simulink model "Pacemaker_01"  (R2020a)
settings: Solver=FixedStepAuto  StartTime=0.0  StopTime=10.0  FixedStep=1e-3  RelTol=1e-3  EnableMultiTasking=on
undefined symbols (not defined in the file): D0, D10, D11, D2, D5, D8, PTA0, PTA2, PTB9, PTC16, PTD0, PTD2
libraries: frdmk64flib x14
settings Model: ExtModeTrigDuration=5  Creator=forre  LastModifiedBy=forre
settings OptimizationCC: EnhancedBackFolding=on  PassReuseOutputArgsAs=Individual arguments  ZeroExternalMemoryAtStartup=off  ZeroInternalMemoryAtStartup=off  MaxStackSize=64  OptimizeBlockOrder=speed  DifferentSizesBufferReuse=on  OptimizationCustomize=off  EfficientTunableParamExpr=on
settings DebuggingCC: ParameterTunabilityLossMsg=error
settings HardwareCC: ProdBitPerPointer=32  ProdBitPerSizeT=32  ProdBitPerPtrDiffT=32  ProdLargestAtomicInteger=Long  ProdLargestAtomicFloat=Double  ProdWordSize=32  ProdHWDeviceType=ARM Compatible->ARM Cortex
settings SFSimCC: MATLABDynamicMemAlloc=off
settings RTWCC: SystemTargetFile=ert.tlc  HardwareBoard=NXP FRDM-K64F  TemplateMakefile=ert_default_tmf  Toolchain=GNU Tools for ARM Embedded Processors
settings CodeAppCC: ForceParamTrailComments=on  IgnoreCustomStorageClasses=off  OperatorAnnotations=on  SimulinkDataObjDesc=on  SFDataObjDesc=on  InsertBlockDesc=on

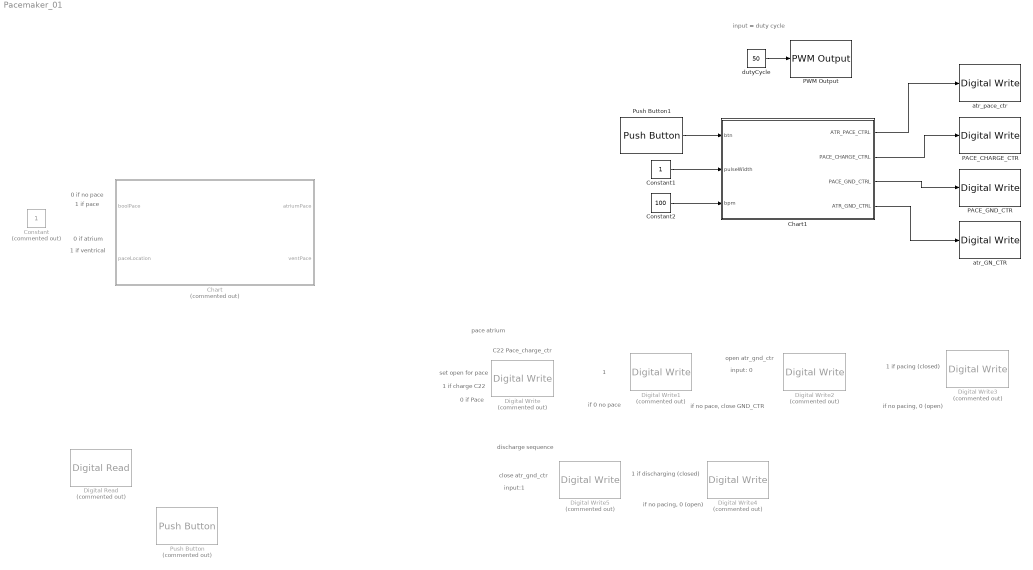
== system Pacemaker_01 ==
  note: 1 if pace
  note: 0 if no pace
  note: 1 if ventrical
  note: 0 if atrium
  note: input = duty cycle
  note: set open for pace
  note: discharge sequence
  note: if no pacing, 0 (open)
  note: 1 if pacing (closed)
  note: if no pace, close GND_CTR
  note: input: 0
  note: open atr_gnd_ctr
  note: if 0 no pace
  note: 1
  note: pace atrium
  note: 0 if Pace
  note: 1 if charge C22
  note: C22 Pace_charge_ctr
  note: if no pacing, 0 (open)
  note: 1 if discharging (closed)
  note: input:1
  note: close atr_gnd_ctr
  Chart : Stateflow chart  Commented=on  TreatAsAtomicUnit=on
  Chart1 : Stateflow chart  TreatAsAtomicUnit=on
  Constant : Constant  Commented=on
  Constant1 : Constant
  Constant2 : Constant  Value=100
  Digital Read : frdmk64flib/Digital Read  Commented=on  Whichpin=PTC16 (D0)  SampleTime=-1
  Digital Write : frdmk64flib/Digital Write  Commented=on  Whichpin=PTB9 (D2)
  Digital Write1 : frdmk64flib/Digital Write  Commented=on  Whichpin=PTA0 (D8)
  Digital Write2 : frdmk64flib/Digital Write  Commented=on  Whichpin=PTD2 (D11)
  Digital Write3 : frdmk64flib/Digital Write  Commented=on  Whichpin=PTD0 (D10)
  Digital Write4 : frdmk64flib/Digital Write  Commented=on  Whichpin=PTD0 (D10)
  Digital Write5 : frdmk64flib/Digital Write  Commented=on  Whichpin=PTD2 (D11)
  PACE_CHARGE_CTR : frdmk64flib/Digital Write  Whichpin=PTB9 (D2)
  PACE_GND_CTR : frdmk64flib/Digital Write  Whichpin=PTD0 (D10)
  PWM Output : frdmk64flib/PWM Output  Whichpin=PTA2 (D5)  InitialFrequency=1000  InitialDutyCycle=50
  Push Button : frdmk64flib/Push Button  Commented=on  Whichswitch=SW2  SampleTime1=-1
  Push Button1 : frdmk64flib/Push Button  Whichswitch=SW2  SampleTime1=-1
  atr_GN_CTR : frdmk64flib/Digital Write  Whichpin=PTD2 (D11)
  atr_pace_ctr : frdmk64flib/Digital Write  Whichpin=PTA0 (D8)
  dutyCycle : Constant  Value=50
  wires:
  dutyCycle/1 -> PWM Output/1
  Push Button1/1 -> Chart1/1(btn)
  Chart1/4(ATR_GND_CTRL) -> atr_GN_CTR/1
  Constant1/1 -> Chart1/2(pulseWidth)
  Chart1/1(ATR_PACE_CTRL) -> atr_pace_ctr/1
  Chart1/2(PACE_CHARGE_CTRL) -> PACE_CHARGE_CTR/1
  Chart1/3(PACE_GND_CTRL) -> PACE_GND_CTR/1
  Constant2/1 -> Chart1/3(bpm)

== stateflow chart Pacemaker_01/Chart1 ==
  note: beats per minute
  state CHARGING_AND_DISCHARGE
    entry:
    PACE_GND_CTRL = true; % 10
    ATR_PACE_CTRL = false;
    ATR_GND_CTRL = true; % 7
    PACE_CHARGE_CTRL = true;
    secPerBeat = 60/bpm;
  state PACING
    entry:
    PACE_GND_CTRL = true; %10
    ATR_PACE_CTRL = true; % 6
    ATR_GND_CTRL = false; %7
  state DISCHARGE [commented out]
    entry:
    ATR_GND_CTR = true; % 7
    ATR_PACE_CTRL = false; % 6
  (default) -> CHARGING_AND_DISCHARGE
  CHARGING_AND_DISCHARGE -> PACING : after(secPerBeat, sec){PACE_CHARGE_CTRL = false;}
  PACING -> CHARGING_AND_DISCHARGE : after(pulseWidth, msec)
  data: btn input boolean; ATR_PACE_CTRL output boolean; PACE_CHARGE_CTRL output boolean; PACE_GND_CTRL output boolean; ATR_GND_CTRL output boolean; pulseWidth input double; bpm input double; secPerBeat local double

== stateflow chart Pacemaker_01/Chart ==
  state ATRIUM_PACE
    entry:
    atriumPace = True;
    ventPace = False;
  state PACE_CTR
    entry:
    ;
  state VENTRICAL_PACE
    entry:
    atriumPace = False;
    ventPace = True;
  (default) -> PACE_CTR
  PACE_CTR -> ATRIUM_PACE [order 1] : [~paceLocation]
  PACE_CTR -> VENTRICAL_PACE [order 2] : [paceLocation]
  data: boolPace input boolean; paceLocation input boolean; atriumPace output boolean; ventPace output boolean
